simulink model "FDMA"  (R2022b)
settings: Solver=VariableStepAuto  StartTime=0.0  StopTime=10.0  RelTol=1e-3
libraries: dsparch4 x4
settings Model: Creator=Admin  LastModifiedBy=Admin

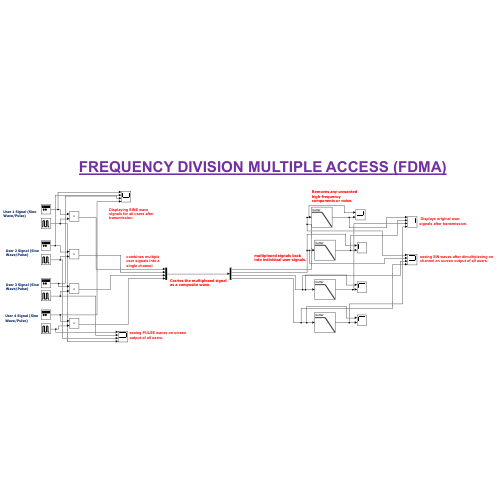
[thumbnail: Simulink's stored preview of the top-level diagram]
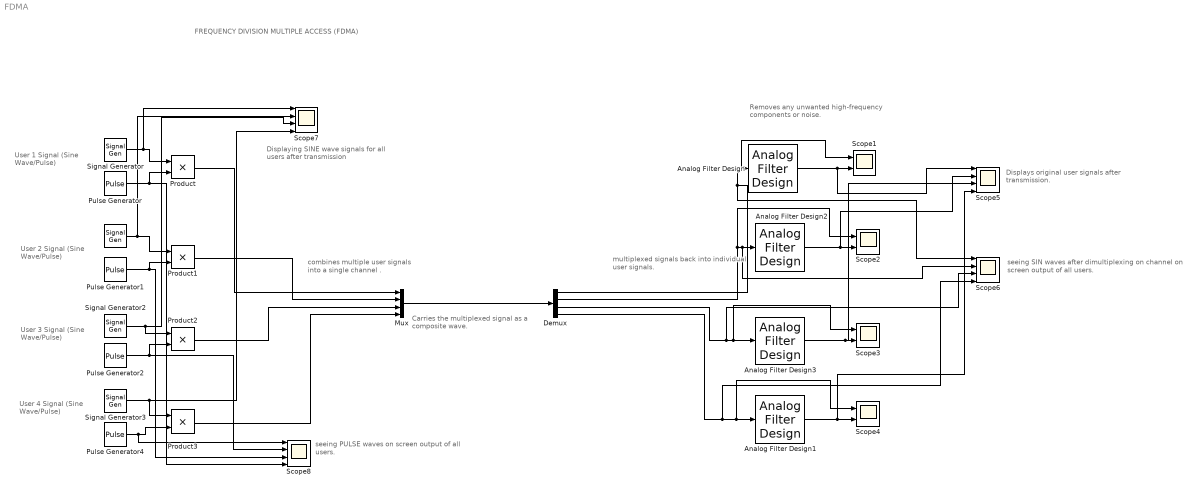
== system FDMA ==
  note: seeing PULSE waves on screen output of all users.
  note: User 1 Signal (Sine Wave/Pulse)
  note: Removes any unwanted high-frequency components or noise.
  note: Carries the multiplexed signal as a composite wave.
  note: Displaying SINE wave signals for all users after transmission
  note: User 4 Signal (Sine Wave/Pulse)
  note: FREQUENCY DIVISION MULTIPLE ACCESS (FDMA)
  note: multiplexed signals back into individual user signals.
  note: combines multiple user signals into a single channel .
  note: Displays original user signals after transmission.
  note: User 3 Signal (Sine Wave/Pulse)
  note: User 2 Signal (Sine Wave/Pulse)
  note: seeing SIN waves after dimultiplexing on channel on screen output of all users.
  " " : SignalGenerator  Frequency=3*pi  Units=rad/sec
  Analog Filter Design{,1..3} (4 alike) : dsparch4/Analog Filter Design  method=Butterworth  filttype=Lowpass  N=8  Wlo=30  Whi=80  Rp=2  Rs=40
  Demux : Demux
  Mux : Mux
  Product{,1..3} (4 alike) : Product
  Pulse Generator{,1..2,4} (4 alike) : DiscretePulseGenerator  PulseType=Time based  Period=0.1  PulseWidth=25
  Scope{1..4} (4 alike) : Scope  NumInputPorts=2
  Scope{5..8} (4 alike) : Scope  NumInputPorts=4
  Signal Generator : SignalGenerator  Frequency=2*pi  Units=rad/sec
  Signal Generator2 : SignalGenerator  Frequency=4*pi  Units=rad/sec
  Signal Generator3 : SignalGenerator  Frequency=5*pi  Units=rad/sec
  wires:
  Demux/1 -> Scope1/1, Analog Filter Design/1, Scope6/1
  Demux/3 -> Scope6/3, Scope3/1, Analog Filter Design3/1
  Demux/4 -> Scope6/4, Scope4/1, Analog Filter Design1/1
  " "/1 -> Scope7/2, Product1/1
  Pulse Generator2/1 -> Scope8/2, Product2/2
  Analog Filter Design1/1 -> Scope5/4, Scope4/2
  Pulse Generator4/1 -> Scope8/1, Product3/2
  Product2/1 -> Mux/3
  Signal Generator2/1 -> Scope7/3, Product2/1
  Mux/1 -> Demux/1
  Product/1 -> Mux/1
  Analog Filter Design2/1 -> Scope5/2, Scope2/2
  Product3/1 -> Mux/4
  Signal Generator/1 -> Scope7/1, Product/1
  Product1/1 -> Mux/2
  Pulse Generator1/1 -> Scope8/3, Product1/2
  Analog Filter Design3/1 -> Scope5/3, Scope3/2
  Analog Filter Design/1 -> Scope5/1, Scope1/2
  Demux/2 -> Scope2/1, Scope6/2, Analog Filter Design2/1
  Signal Generator3/1 -> Scope7/4, Product3/1
  Pulse Generator/1 -> Scope8/4, Product/2
